simulink model "AB"  (R2023a)
settings: Solver=FixedStepDiscrete  StartTime=0.0  StopTime=inf  RelTol=1e-3
settings Model: Creator=proto  LastModifiedBy=proto
settings RTWCC: GenerateReport=on  LaunchReport=on
settings GRTTargetCC: UtilityFuncGeneration=Shared location  CodeInterfacePackaging=Reusable function  GenerateAllocFcn=on  RTWCAPISignals=on

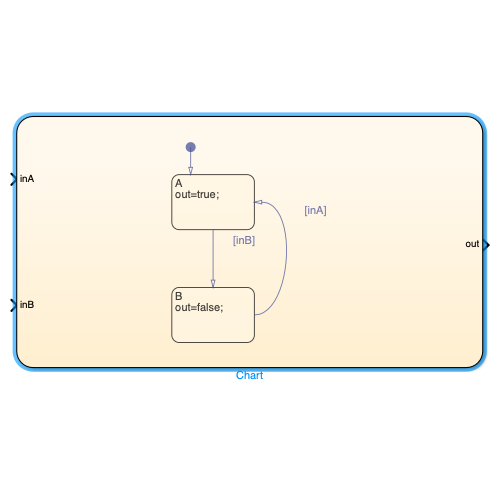
[thumbnail: Simulink's stored preview of the top-level diagram]
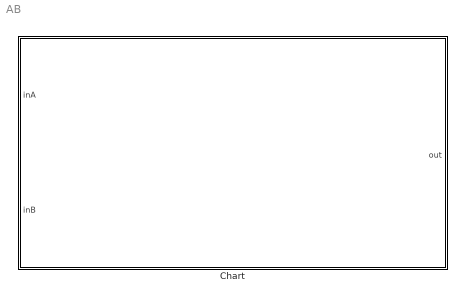
== system AB ==
  Chart : Stateflow chart  TreatAsAtomicUnit=on

== stateflow chart AB/Chart ==
  state A
    out=true;
  state B
    out=false;
  (default) -> A
  B -> A : [inA]
  A -> B : [inB]
  data: inA input boolean size=1; out output boolean size=1; inB input boolean size=1
